simulink model "MassSpringMod"  (R2023b)
settings: Solver=FixedStepAuto  StartTime=0.0  StopTime=100  FixedStep=1  RelTol=1e-3
undefined symbols (not defined in the file): dampingCoefficient, mass, springConstant
settings Model: ExtModeTrigDuration=100  Creator=20181234  LastModifiedBy=20181234
settings DataIOCC: StateSaveName=tmp_raccel_xout
settings OptimizationCC: EfficientMapNaN2IntZero=off
settings DebuggingCC: ModelReferenceSymbolNameMessage=none
settings HardwareCC: TargetBitPerPointer=64  TargetBitPerSizeT=64  TargetBitPerPtrDiffT=64  TargetLongLongMode=on  TargetIntDivRoundTo=Zero  TargetEndianess=LittleEndian  TargetWordSize=64  TargetHWDeviceType=MATLAB Host  ProdEqTarget=off
settings RTWCC: SystemTargetFile=raccel.tlc  TemplateMakefile=raccel_default_tmf  RTWVerbose=off  RTWUseSimCustomCode=on  CustomBLASCallback=coder.internal.blas.MATLABBLASCallback
settings CodeAppCC: GenerateComments=off  MaxIdLength=128  MangleLength=10  SimulinkBlockComments=off
settings RaccelTargetCC: TargetLangStandard=C99 (ISO)  OptimizeReductions=off  ENABLE_SLEXEC_SSBRIDGE=1  RTWCAPIParams=on  RTWCAPIRootIO=on

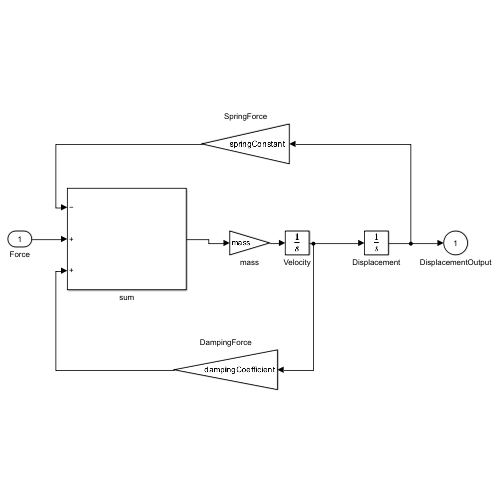
[thumbnail: Simulink's stored preview of the top-level diagram]
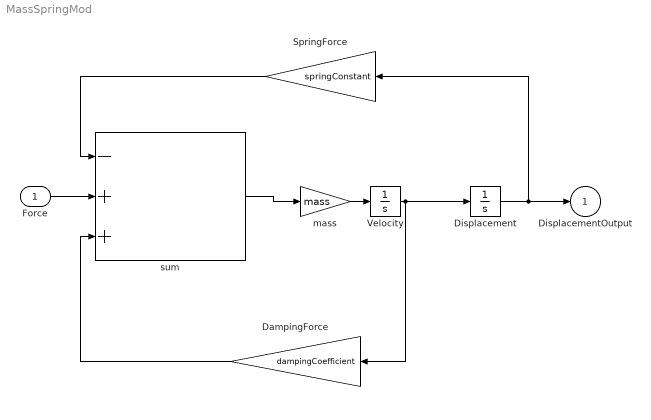
== system MassSpringMod ==
  Force : Inport
  DampingForce : Gain  Gain=dampingCoefficient
  Displacement : Integrator
  SpringForce : Gain  Gain=springConstant
  Velocity : Integrator
  mass : Gain  Gain=mass
  sum : Sum  Inputs=-++
  DisplacementOutput : Outport
  wires:
  Force/1 -> sum/2
  Displacement/1 -> SpringForce/1, DisplacementOutput/1
  SpringForce/1 -> sum/1
  Velocity/1 -> DampingForce/1, Displacement/1
  DampingForce/1 -> sum/3
  sum/1 -> mass/1
  mass/1 -> Velocity/1
